simulink model "Iek1NoActions"  (Simulink 9.0)
settings: Solver=FixedStepDiscrete  StartTime=0.0  StopTime=10000000.0  RelTol=1e-3  EnableMultiTasking=on
settings Model: SuppressorTable=22 serialization::archive 11 0 6 0 0 0 0 0  Creator=scaife  LastModifiedBy=ktrinh  ExtModeAutoUpdateStatusClock=off
settings DataIOCC: LimitDataPoints=on  SignalLoggingSaveFormat=ModelDataLogs  SignalLoggingName=sigsOut
settings DebuggingCC: SaveWithParameterizedLinksMsg=none  SignalResolutionControl=TryResolveAllWithWarning  MultiTaskDSMMsg=warning  MultiTaskCondExecSysMsg=none  StrictBusMsg=None
settings HardwareCC: TargetUnknown=on
settings SFSimCC: SimParseCustomCode=off
settings GRTTargetCC: CombineOutputUpdateFcns=off  GRTInterface=on

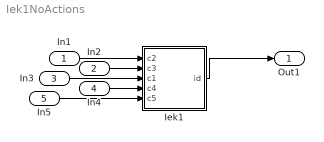
== system Iek1NoActions ==
  In1 : Inport  OutDataTypeStr=boolean
  In2 : Inport  Port=2  OutDataTypeStr=boolean
  In3 : Inport  Port=3  OutDataTypeStr=boolean
  In4 : Inport  Port=4  OutDataTypeStr=boolean
  In5 : Inport  Port=5  OutDataTypeStr=boolean
  Iek1 : Stateflow chart  TreatAsAtomicUnit=on
  Out1 : Outport
  wires:
  Iek1/1(id) -> Out1/1
  In2/1 -> Iek1/2(c3)
  In1/1 -> Iek1/1(c2)
  In3/1 -> Iek1/3(c1)
  In4/1 -> Iek1/4(c4)
  In5/1 -> Iek1/5(c5)

== stateflow chart Iek1 ==
  state T1 [parallel]
    settings: executionOrder=1
    state B
      en: id=2;
    state A
      en: id=1;
    (default) -> A
    B -> A : [c1]
    A -> B : [c1]
  state T2 [parallel]
    settings: executionOrder=2
    state C
      en: id=3;
    state D
      en: id=4
    (default) -> C
    D -> C : [c2]
    C -> D : [c2]
  state T3 [parallel]
    settings: executionOrder=3
    state a
      en: id=7;
    state c
      en: id=8;
    state b
      en: id=6;
    state d
      en: id=5;
    (default) -> a
    a -> c : [c2]
    b -> c [order 2] : [c3]
    b -> a [order 1] : [c5]
    c -> b [order 2] : [c4]
    c -> d [order 1] : [c1]
    d -> b : [c5]
  data: c2 input boolean; c3 input boolean; id output double; c1 input boolean; c4 input boolean; c5 input boolean
